simulink model "reference_signal"  (R2023a)
settings: configuration reference "config" (kept outside this file)
libraries: servo_hub_lib x1
settings Model: DataDictionary=model_config.sldd  Creator=huangcheng  LastModifiedBy=Administrator
settings ConfigSetRef: SourceName=config

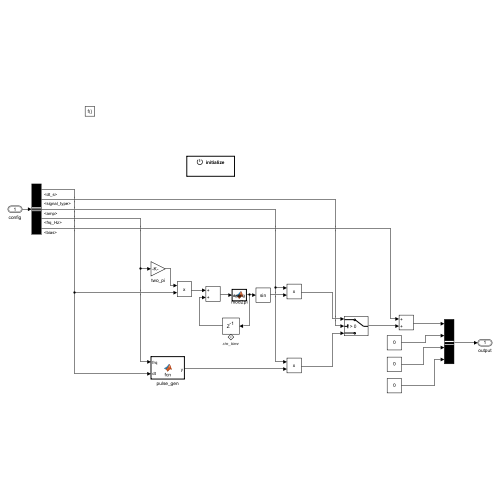
[thumbnail: Simulink's stored preview of the top-level diagram]
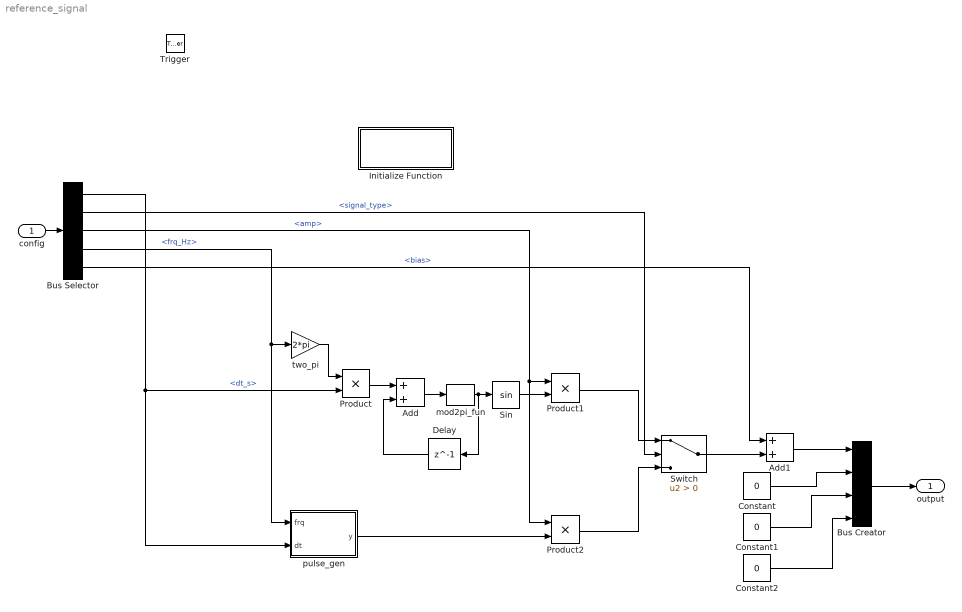
== system reference_signal ==
  config : Inport  OutDataTypeStr=Bus: ReferenceSignalConfig  BusOutputAsStruct=on
  Trigger : TriggerPort  TriggerType=function-call  VariantControl=(inherit)  PortDimensions=1
  Add : Sum
  Add1 : Sum
  Bus Creator : BusCreator  Inputs=4  OutDataTypeStr=Bus: ReferenceSignalOutput  NonVirtualBus=on
      settings: InheritFromInputs=off
  Bus Selector : BusSelector  OutputSignals=dt_s,signal_type,amp,frq_Hz,bias
  Constant : Constant  Value=0  OutDataTypeStr=int64
  Constant1 : Constant  Value=0  OutDataTypeStr=single
  Constant2 : Constant  Value=0  OutDataTypeStr=single
  Delay : Delay  DelayLength=1  StateName=sin_time
  Initialize Function : Subsystem  TreatAsAtomicUnit=on
  Product : Product
  Product1 : Product
  Product2 : Product
  Sin : Trigonometry
  Switch : Switch  Criteria=u2 > Threshold  SaturateOnIntegerOverflow=off  InputSameDT=off
  mod2pi_fun : servo_hub_lib/fast_math/mod2pi_fun  SystemSampleTime=-1  VariantActivationTime=update diagram  Latency=0  AutoFrameSizeCalculation=off
      settings: LibrarySourceBlock=|
      | simulink/User-Defined
      | Functions/MATLAB Function
  pulse_gen : MATLAB Function  TreatAsAtomicUnit=on
  two_pi : Gain  Gain=2*pi
  output : Outport  OutDataTypeStr=Bus: ReferenceSignalOutput  BusOutputAsStruct=on
  wires:
  Bus Selector/2 -> Switch/2  "<signal_type>"
  Bus Selector/1 -> pulse_gen/2(dt), Product/2  "<dt_s>"
  Delay/1 -> Add/2
  two_pi/1 -> Product/1
  Sin/1 -> Product1/2
  Product1/1 -> Switch/1
  pulse_gen/1(y) -> Product2/2
  Product2/1 -> Switch/3
  Switch/1 -> Add1/2
  Add1/1 -> Bus Creator/1
  Bus Creator/1 -> output/1
  config/1 -> Bus Selector/1
  Bus Selector/3 -> Product1/1, Product2/1  "<amp>"
  Bus Selector/4 -> pulse_gen/1(frq), two_pi/1  "<frq_Hz>"
  Bus Selector/5 -> Add1/1  "<bias>"
  Product/1 -> Add/1
  Add/1 -> mod2pi_fun/1
  mod2pi_fun/1 -> Delay/1, Sin/1
  Constant/1 -> Bus Creator/2
  Constant1/1 -> Bus Creator/3
  Constant2/1 -> Bus Creator/4

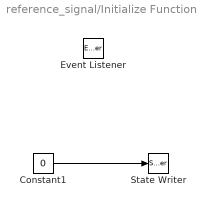
== system reference_signal/Initialize Function ==
  Constant1 : Constant  Value=0  OutDataTypeStr=single
  Event Listener : EventListener  DisableCoverage=on  EventName=reset
  State Writer : StateWriter  StateOwnerBlock=../../Delay  StateName=sin_time
  wires:
  Constant1/1 -> State Writer/1

== matlab function reference_signal/pulse_gen ==
  data: frq input; dt input; y output
function y = fcn(frq, dt)

persistent times;

if isempty(times)
    times = single(0);
end

time_out = single(1.0)/frq;
half_time_out = single(0.5) * time_out;

if times >= time_out
    times = single(0);
end

times = times + dt;


if times > half_time_out
    y = single(1);
else
    y = single(0);
end
